simulink model "untitled"  (Simulink 9.2)
settings: Solver=ode45  StartTime=0.0  StopTime=50  RelTol=1e-3  EnableMultiTasking=on
undefined symbols (not defined in the file or in its folder): DiscIntNeverNeededParam, Kd, Ki, Kp
settings Model: Creator=Administrator  LastModifiedBy=ILQMN
settings DataIOCC: SignalLoggingSaveFormat=Dataset
settings DebuggingCC: UnderspecifiedInitializationDetection=Simplified  MergeDetectMultiDrivingBlocksExec=error  SolverPrmCheckMsg=warning  FcnCallInpInsideContextMsg=error  AllowSymbolicDim=off  StateNameClashWarn=none
settings GRTTargetCC: CombineOutputUpdateFcns=on  GRTInterface=off
settings ConfigComp: CovSFcnEnable=off

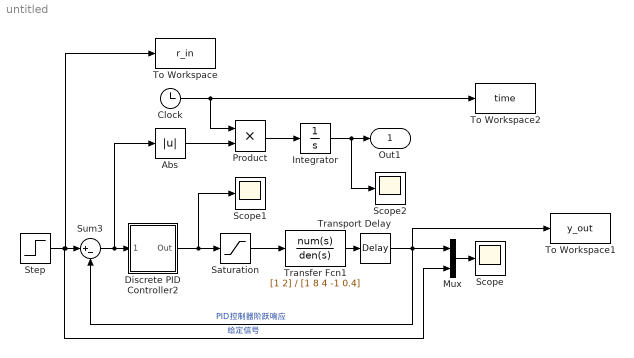
== system untitled ==
  Abs : Abs
  Clock : Clock
  Discrete PID Controller2 : Subsystem  AncestorBlock=|  DialogController=POWERSYS.PowerSysDialog  mask(Discrete PID Controller){Kp=Kp, Ki=Ki, Kd=Kd, TcD=0.5, Par_Limits=[10 0], Init=0, Ts=0.5}
      | powerlib_extras/Discrete 
      | Control Blocks/Discrete
      | PID Controller
      mask prompts: Kp "Proportional gain (Kp):"; Ki "Integral gain (Ki):"; Kd "Derivative gain (Kd):"; TcD "Time constant for derivative (s):"; Par_Limits "Output limits: [ Upper   Lower ]"; Init "Output initial value:"; Ts "Sample time:"
      mask help: This block implements a discrete PID controller.
      mask init:
      | UpperLimit=Par_Limits(1);
      | LowerLimit=Par_Limits(2);
      | power_initmask();
      mask Help: This block is part of a subset of blocks in the Extras library that does not have documentation associated with it, other than the block mask description.
      mask Display: disp('PID');
  Integrator : Integrator
  Mux : Mux  Inputs=2
  Product : Product
  Saturation : Saturate  UpperLimit=10
  Scope : Scope
  Scope1 : Scope
  Scope2 : Scope
  Step : Step  Time=0  Before=1  SampleTime=0
  Sum3 : Sum  Inputs=|+-
  To Workspace : ToWorkspace  VariableName=r_in  SampleTime=0.1
  To Workspace1 : ToWorkspace  VariableName=y_out  SampleTime=0.1
  To Workspace2 : ToWorkspace  VariableName=time  SampleTime=0.1
  Transfer Fcn1 : TransferFcn  Numerator=[1 2]  Denominator=[1 8 4 -1 0.4]
  Transport Delay : TransportDelay  DelayTime=3
  Out1 : Outport
  wires:
  Transfer Fcn1/1 -> Transport Delay/1
  Transport Delay/1 -> To Workspace1/1, Mux/1, Sum3/2  "PID控制器阶跃响应"
  Discrete PID Controller2/1(Out) -> Saturation/1, Scope1/1
  Sum3/1 -> Abs/1, Discrete PID Controller2/1(Error)
  Step/1 -> Mux/2, To Workspace/1, Sum3/1  "给定信号"
  Abs/1 -> Product/2
  Clock/1 -> To Workspace2/1, Product/1
  Product/1 -> Integrator/1
  Integrator/1 -> Scope2/1, Out1/1
  Mux/1 -> Scope/1
  Saturation/1 -> Transfer Fcn1/1

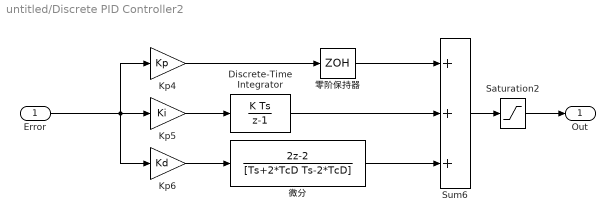
== system untitled/Discrete PID Controller2 ==
  Error : Inport  SampleTime=Ts
  Discrete-Time Integrator : DiscreteIntegrator  InitialCondition=Init  SampleTime=Ts  LimitOutput=on  UpperSaturationLimit=UpperLimit  LowerSaturationLimit=LowerLimit  ICPrevOutput=DiscIntNeverNeededParam  ICPrevScaledInput=DiscIntNeverNeededParam
  Kp4 : Gain  Gain=Kp  SampleTime=Ts  SaturateOnIntegerOverflow=on  OutDataTypeStr=Inherit: Same as input  ParamDataTypeStr=Inherit: Same as input
  Kp5 : Gain  Gain=Ki  SampleTime=Ts  SaturateOnIntegerOverflow=on  OutDataTypeStr=Inherit: Same as input  ParamDataTypeStr=Inherit: Same as input
  Kp6 : Gain  Gain=Kd  SampleTime=Ts  SaturateOnIntegerOverflow=on  OutDataTypeStr=Inherit: Same as input  ParamDataTypeStr=Inherit: Same as input
  Saturation2 : Saturate  UpperLimit=UpperLimit  LowerLimit=LowerLimit  SampleTime=Ts
  Sum6 : Sum  Inputs=+++  SampleTime=Ts  SaturateOnIntegerOverflow=on  InputSameDT=on  OutDataTypeStr=Inherit: Same as first input
  "微分 " : DiscreteTransferFcn  Numerator=[2 -2]  Denominator=[Ts+2*TcD Ts-2*TcD]  SampleTime=Ts
  零阶保持器 : ZeroOrderHold  SampleTime=Ts
  Out : Outport  SampleTime=Ts  InitialOutput=0
  wires:
  Saturation2/1 -> Out/1
  Error/1 -> Kp4/1, Kp5/1, Kp6/1
  Sum6/1 -> Saturation2/1
  Kp5/1 -> Discrete-Time Integrator/1
  Kp6/1 -> "微分 "/1
  Kp4/1 -> 零阶保持器/1
  Discrete-Time Integrator/1 -> Sum6/2
  "微分 "/1 -> Sum6/3
  零阶保持器/1 -> Sum6/1
